simulink model "LFAST_System"  (R2022b)
settings: Solver=VariableStepAuto  StartTime=0.0  StopTime=10.0  RelTol=1e-3
model workspace (MAT data in the model file):
  LFAST_TCP_Comms = Simulink.Bus
  LFAST_TCP_Comms.Alignment = -1
  LFAST_TCP_Comms.PreserveElementDimensions = 0
  LFAST_TCP_Comms.DataScope = 'Auto'
  Modbus = Simulink.Bus
  Modbus.Alignment = -1
  Modbus.PreserveElementDimensions = 0
  Modbus.Elements_internal(1) = Simulink.BusElement
  Modbus.Elements_internal(1).DimensionsMode = 'Fixed'
  Modbus.Elements_internal(1).SamplingMode = 'Sample based'
  Modbus.Elements_internal(1).SampleTime = -1
  Modbus.Elements_internal(1).Name = 'Slave_ID'
  Modbus.Elements_internal(1).DataType_internal = 'double'
  Modbus.Elements_internal(1).Complexity = 'real'
  Modbus.Elements_internal(1).Dimensions = 1
  Modbus.Elements_internal(2) = Simulink.BusElement
  Modbus.Elements_internal(2).DimensionsMode = 'Fixed'
  Modbus.Elements_internal(2).SamplingMode = 'Sample based'
  Modbus.Elements_internal(2).SampleTime = -1
  Modbus.Elements_internal(2).Name = 'CONTROL_WORD'
  Modbus.Elements_internal(2).DataType_internal = 'double'
  Modbus.Elements_internal(2).Complexity = 'real'
  Modbus.Elements_internal(2).Dimensions = 1
  Modbus.Elements_internal(3) = Simulink.BusElement
  Modbus.Elements_internal(3).DimensionsMode = 'Fixed'
  Modbus.Elements_internal(3).SamplingMode = 'Sample based'
  Modbus.Elements_internal(3).SampleTime = -1
  Modbus.Elements_internal(3).Name = 'STATUS_WORD'
  Modbus.Elements_internal(3).DataType_internal = 'double'
  Modbus.Elements_internal(3).Complexity = 'real'
  Modbus.Elements_internal(3).Dimensions = 1
  Modbus.Elements_internal(4) = Simulink.BusElement
  Modbus.Elements_internal(4).DimensionsMode = 'Fixed'
  Modbus.Elements_internal(4).SamplingMode = 'Sample based'
  Modbus.Elements_internal(4).SampleTime = -1
  Modbus.Elements_internal(4).Name = 'OPERATION_MODE'
  Modbus.Elements_internal(4).DataType_internal = 'double'
  Modbus.Elements_internal(4).Complexity = 'real'
  Modbus.Elements_internal(4).Dimensions = 1
  Modbus.Elements_internal(5) = Simulink.BusElement
  Modbus.Elements_internal(5).DimensionsMode = 'Fixed'
  Modbus.Elements_internal(5).SamplingMode = 'Sample based'
  Modbus.Elements_internal(5).SampleTime = -1
  Modbus.Elements_internal(5).Name = 'ABS_REL_SELECT'
  Modbus.Elements_internal(5).DataType_internal = 'double'
  Modbus.Elements_internal(5).Complexity = 'real'
  Modbus.Elements_internal(5).Dimensions = 1
  Modbus.Elements_internal(6) = Simulink.BusElement
  Modbus.Elements_internal(6).DimensionsMode = 'Fixed'
  Modbus.Elements_internal(6).SamplingMode = 'Sample based'
  Modbus.Elements_internal(6).SampleTime = -1
  Modbus.Elements_internal(6).Name = 'POS_ACTUAL'
  Modbus.Elements_internal(6).DataType_internal = 'double'
  Modbus.Elements_internal(6).Complexity = 'real'
  Modbus.Elements_internal(6).Dimensions = 1
  Modbus.Elements_internal(7) = Simulink.BusElement
  Modbus.Elements_internal(7).DimensionsMode = 'Fixed'
  Modbus.Elements_internal(7).SamplingMode = 'Sample based'
  Modbus.Elements_internal(7).SampleTime = -1
  Modbus.Elements_internal(7).Name = 'REAL_CURRENT'
  Modbus.Elements_internal(7).DataType_internal = 'double'
  Modbus.Elements_internal(7).Complexity = 'real'
  Modbus.Elements_internal(7).Dimensions = 1
  Modbus.Elements_internal(8) = Simulink.BusElement
  Modbus.Elements_internal(8).DimensionsMode = 'Fixed'
  Modbus.Elements_internal(8).SamplingMode = 'Sample based'
  Modbus.Elements_internal(8).SampleTime = -1
  Modbus.Elements_internal(8).Name = 'REAL_SPEED'
  Modbus.Elements_internal(8).DataType_internal = 'double'
  Modbus.Elements_internal(8).Complexity = 'real'
  Modbus.Elements_internal(8).Dimensions = 1
  Modbus.Elements_internal(9) = Simulink.BusElement
  Modbus.Elements_internal(9).DimensionsMode = 'Fixed'
  Modbus.Elements_internal(9).SamplingMode = 'Sample based'
  Modbus.Elements_internal(9).SampleTime = -1
  Modbus.Elements_internal(9).Name = 'TARGET_POS'
  Modbus.Elements_internal(9).DataType_internal = 'double'
  Modbus.Elements_internal(9).Complexity = 'real'
  Modbus.Elements_internal(9).Dimensions = 1
  Modbus.Elements_internal(10) = Simulink.BusElement
  Modbus.Elements_internal(10).DimensionsMode = 'Fixed'
  Modbus.Elements_internal(10).SamplingMode = 'Sample based'
  Modbus.Elements_internal(10).SampleTime = -1
  Modbus.Elements_internal(10).Name = 'PROFILE_SPEED'
  Modbus.Elements_internal(10).DataType_internal = 'double'
  Modbus.Elements_internal(10).Complexity = 'real'
  Modbus.Elements_internal(10).Dimensions = 1
  Modbus.Elements_internal(11) = Simulink.BusElement
  Modbus.Elements_internal(11).DimensionsMode = 'Fixed'
  Modbus.Elements_internal(11).SamplingMode = 'Sample based'
  Modbus.Elements_internal(11).SampleTime = -1
  Modbus.Elements_internal(11).Name = 'TARGET_SPEED'
  Modbus.Elements_internal(11).DataType_internal = 'double'
  Modbus.Elements_internal(11).Complexity = 'real'
  Modbus.Elements_internal(11).Dimensions = 1
  Modbus.Elements_internal(12) = Simulink.BusElement
  Modbus.Elements_internal(12).DimensionsMode = 'Fixed'
  Modbus.Elements_internal(12).SamplingMode = 'Sample based'
  Modbus.Elements_internal(12).SampleTime = -1
  Modbus.Elements_internal(12).Name = 'MAX_SPEED'
  Modbus.Elements_internal(12).DataType_internal = 'double'
  Modbus.Elements_internal(12).Complexity = 'real'
  Modbus.Elements_internal(12).Dimensions = 1
  Modbus.Elements_internal(13) = Simulink.BusElement
  Modbus.Elements_internal(13).DimensionsMode = 'Fixed'
  Modbus.Elements_internal(13).SamplingMode = 'Sample based'
  Modbus.Elements_internal(13).SampleTime = -1
  Modbus.Elements_internal(13).Name = 'PROFILE_ACC'
  Modbus.Elements_internal(13).DataType_internal = 'double'
  Modbus.Elements_internal(13).Complexity = 'real'
  Modbus.Elements_internal(13).Dimensions = 1
  Modbus.Elements_internal(14) = Simulink.BusElement
  Modbus.Elements_internal(14).DimensionsMode = 'Fixed'
  Modbus.Elements_internal(14).SamplingMode = 'Sample based'
  Modbus.Elements_internal(14).SampleTime = -1
  Modbus.Elements_internal(14).Name = 'PROFILE_DEC'
  Modbus.Elements_internal(14).DataType_internal = 'double'
  Modbus.Elements_internal(14).Complexity = 'real'
  Modbus.Elements_internal(14).Dimensions = 1
  Modbus.Elements_internal(15) = Simulink.BusElement
  Modbus.Elements_internal(15).DimensionsMode = 'Fixed'
  Modbus.Elements_internal(15).SamplingMode = 'Sample based'
  Modbus.Elements_internal(15).SampleTime = -1
  Modbus.Elements_internal(15).Name = 'TARGET_TRQ'
  Modbus.Elements_internal(15).DataType_internal = 'double'
  Modbus.Elements_internal(15).Complexity = 'real'
  Modbus.Elements_internal(15).Dimensions = 1
  Modbus.DataScope = 'Auto'
undefined symbols (not defined in the file): AlignmentSubsystem, GuiderInterface, INDI, MessageIn, MessageOut, Telescope
settings Model: Creator=keving  LastModifiedBy=kevin
settings ModelReferenceCC: EnableRefExpFcnMdlSchedulingChecks=on

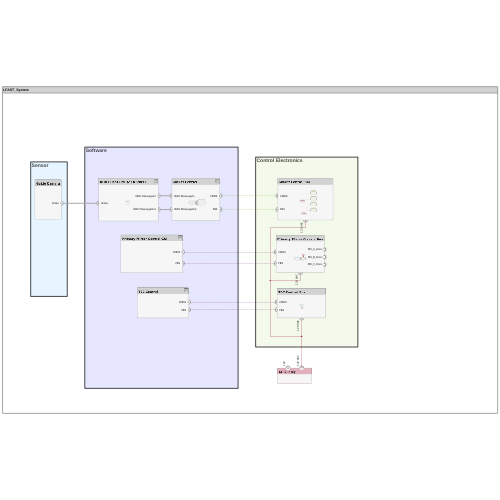
[thumbnail: Simulink's stored preview of the top-level diagram]
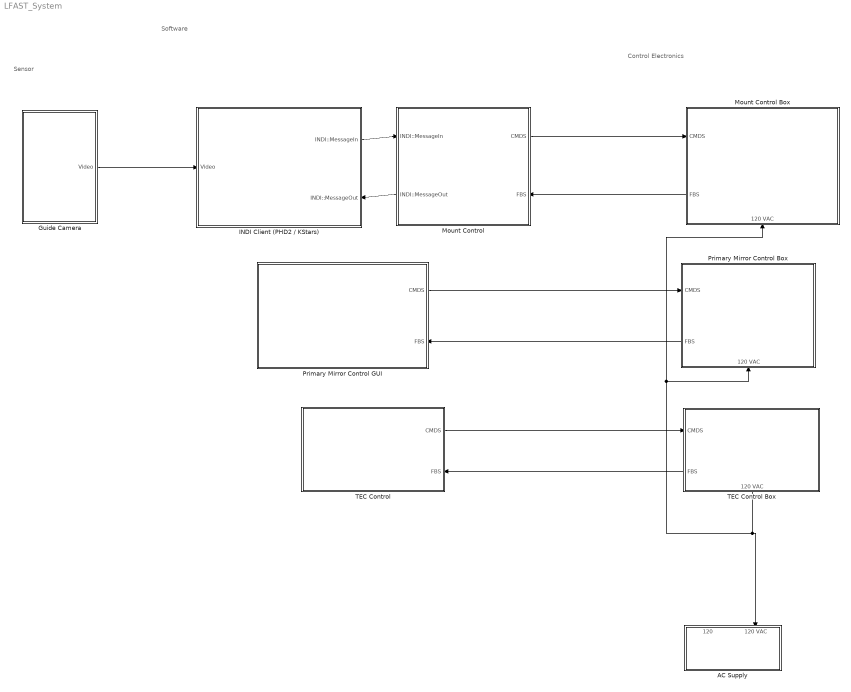
== system LFAST_System ==
  note: Sensor
  note: Software
  note: Control Electronics
  AC Supply : Subsystem
      settings: PortSchema="{\"entries\":[{\"content\":{\"headerSize\":26,\"margin\":15,\"minimumSpacing\":25,\"sides\":[{\"content\":{\"connectorIds\":[]},\"type\":\"ConnectorPlacement.EquallySpacedRectSide\",\"uuid\":\"98751f74-1494-480e-afcb-1e4ca4833d8c\"},{\"content\":{\"connectorIds\":[],\"side\":\"RIGHT\"},\"type\":\"ConnectorPlacement.EquallySpacedRectSide\",\"uuid\":\"bb8add54-8697-4b5a-a683-6c55bc29b1b0\"},{\"content\":{\"connectorIds\":[\"Out1\",\"In1\"],\"side\":\"TOP\"},\"type\":\"ConnectorPlacement.EquallySpacedRectSide\",\"uuid\":\"300d0c82-b670-4163-bf95-251aaf6b9511\"},{\"content\":{\"connectorIds\":[],\"side\":\"BOTTOM\"},\"type\":\"ConnectorPlacement.EquallySpacedRectSide\",\"uuid\":\"167ec2d4-c810-4164-afac-a7cf55661aff\"}]},\"type\":\"ConnectorPlacement.EquallySpacedConnector\",\"uuid\":\"bf69df94-f6ab-4503-8752-ba9a09e2aadb\"}],\"packageUris\":[\"http://schema.mathworks.com/mf0/Connector/R2020b\"],\"version\":\"1.0\"}"
  Guide Camera : Subsystem
      settings: PortSchema="{\"entries\":[{\"content\":{\"headerSize\":26,\"margin\":15,\"minimumSpacing\":25,\"sides\":[{\"content\":{\"connectorIds\":[]},\"type\":\"ConnectorPlacement.EquallySpacedRectSide\",\"uuid\":\"16df8581-7966-4d2c-895b-cc4ea5e246e2\"},{\"content\":{\"connectorIds\":[\"Out1\"],\"side\":\"RIGHT\"},\"type\":\"ConnectorPlacement.EquallySpacedRectSide\",\"uuid\":\"5d59704d-ff3e-44f0-a7f2-847c95827cea\"},{\"content\":{\"connectorIds\":[],\"side\":\"TOP\"},\"type\":\"ConnectorPlacement.EquallySpacedRectSide\",\"uuid\":\"ec3ed101-a96e-4d79-89e3-2afa312ea215\"}]},\"type\":\"ConnectorPlacement.EquallySpacedConnector\",\"uuid\":\"5d368a71-4eba-4adc-b01b-0abb6bcb9ebc\"}],\"packageUris\":[\"http://schema.mathworks.com/mf0/Connector/R2020b\"],\"version\":\"1.0\"}"
  INDI Client (PHD2 / KStars) : Subsystem
      settings: PortSchema="{\"entries\":[{\"content\":{\"headerSize\":26,\"margin\":15,\"minimumSpacing\":25,\"sides\":[{\"content\":{\"connectorIds\":[\"In1\"]},\"type\":\"ConnectorPlacement.EquallySpacedRectSide\",\"uuid\":\"1ee64d24-9451-4e89-96b0-c6c86ed53331\"},{\"content\":{\"connectorIds\":[\"Out1\",\"In2\"],\"side\":\"RIGHT\"},\"type\":\"ConnectorPlacement.EquallySpacedRectSide\",\"uuid\":\"58644688-a0cb-4784-bb9d-85cd24f76786\"},{\"content\":{\"connectorIds\":[],\"side\":\"TOP\"},\"type\":\"ConnectorPlacement.EquallySpacedRectSide\",\"uuid\":\"73e421bb-b1b1-4cf2-a19d-6b2642b6c763\"},{\"content\":{\"connectorIds\":[],\"side\":\"BOTTOM\"},\"type\":\"ConnectorPlacement.EquallySpacedRectSide\",\"uuid\":\"a1df0027-ba85-456a-a33c-a4e3aae0142d\"}]},\"type\":\"ConnectorPlacement.EquallySpacedConnector\",\"uuid\":\"5578c5ac-9f78-4996-ba84-f029b9b17e19\"}],\"packageUris\":[\"http://schema.mathworks.com/mf0/Connector/R2020b\"],\"version\":\"1.0\"}"
  Mount Control : Subsystem
      settings: PortSchema="{\"entries\":[{\"content\":{\"headerSize\":26,\"margin\":15,\"minimumSpacing\":25,\"sides\":[{\"content\":{\"connectorIds\":[\"In2\",\"Out2\"]},\"type\":\"ConnectorPlacement.EquallySpacedRectSide\",\"uuid\":\"1e7a6f7e-04b1-487d-9c42-3f004f45fff7\"},{\"content\":{\"connectorIds\":[\"Out1\",\"In1\"],\"side\":\"RIGHT\"},\"type\":\"ConnectorPlacement.EquallySpacedRectSide\",\"uuid\":\"1d40cd5a-d50e-48bb-ba62-29f418ee0b7d\"},{\"content\":{\"connectorIds\":[],\"side\":\"TOP\"},\"type\":\"ConnectorPlacement.EquallySpacedRectSide\",\"uuid\":\"8c60b213-5e96-4c1f-bace-a9a184d6d43c\"},{\"content\":{\"connectorIds\":[],\"side\":\"BOTTOM\"},\"type\":\"ConnectorPlacement.EquallySpacedRectSide\",\"uuid\":\"7f5ded68-ba2c-42b9-9d6b-2756d3ededc8\"}]},\"type\":\"ConnectorPlacement.EquallySpacedConnector\",\"uuid\":\"740ba7aa-7f0b-4fdf-8ac9-38c1be24b304\"}],\"packageUris\":[\"http://schema.mathworks.com/mf0/Connector/R2020b\"],\"version\":\"1.0\"}"
  Mount Control Box : Subsystem
      settings: PortSchema="{\"entries\":[{\"content\":{\"headerSize\":26,\"margin\":15,\"minimumSpacing\":25,\"sides\":[{\"content\":{\"connectorIds\":[\"In2\",\"Out1\"]},\"type\":\"ConnectorPlacement.EquallySpacedRectSide\",\"uuid\":\"16df8581-7966-4d2c-895b-cc4ea5e246e2\"},{\"content\":{\"connectorIds\":[],\"side\":\"RIGHT\"},\"type\":\"ConnectorPlacement.EquallySpacedRectSide\",\"uuid\":\"5d59704d-ff3e-44f0-a7f2-847c95827cea\"},{\"content\":{\"connectorIds\":[],\"side\":\"TOP\"},\"type\":\"ConnectorPlacement.EquallySpacedRectSide\",\"uuid\":\"ec3ed101-a96e-4d79-89e3-2afa312ea215\"},{\"content\":{\"connectorIds\":[\"In1\"],\"side\":\"BOTTOM\"},\"type\":\"ConnectorPlacement.EquallySpacedRectSide\",\"uuid\":\"65d70669-a716-492b-bf91-097d7de9987f\"}]},\"type\":\"ConnectorPlacement.EquallySpacedConnector\",\"uuid\":\"5d368a71-4eba-4adc-b01b-0abb6bcb9ebc\"}],\"packageUris\":[\"http://schema.mathworks.com/mf0/Connector/R2020b\"],\"version\":\"1.0\"}"
  Primary Mirror Control Box : Subsystem
      settings: PortSchema="{\"entries\":[{\"content\":{\"headerSize\":26,\"margin\":15,\"minimumSpacing\":25,\"sides\":[{\"content\":{\"connectorIds\":[\"In2\",\"Out1\"]},\"type\":\"ConnectorPlacement.EquallySpacedRectSide\",\"uuid\":\"8068dc4f-e0e9-4f1b-946a-b531e46fc784\"},{\"content\":{\"connectorIds\":[\"RConn1\",\"RConn2\",\"RConn3\"],\"side\":\"RIGHT\"},\"type\":\"ConnectorPlacement.EquallySpacedRectSide\",\"uuid\":\"7b44236b-1168-43b8-b2b4-5e873209dfa3\"},{\"content\":{\"connectorIds\":[],\"side\":\"TOP\"},\"type\":\"ConnectorPlacement.EquallySpacedRectSide\",\"uuid\":\"fca4122f-6519-48a9-876a-2e597a8d3bc7\"},{\"content\":{\"connectorIds\":[\"In1\"],\"side\":\"BOTTOM\"},\"type\":\"ConnectorPlacement.EquallySpacedRectSide\",\"uuid\":\"6f4aa163-7b47-4691-94b1-15c4b7706454\"}]},\"type\":\"ConnectorPlacement.EquallySpacedConnector\",\"uuid\":\"9787fa30-fe20-4a09-9d69-8b8b4a760450\"}],\"packageUris\":[\"http://schema.mathworks.com/mf0/Connector/R2020b\"],\"version\":\"1.0\"}"
  Primary Mirror Control GUI : Subsystem
      settings: PortSchema="{\"entries\":[{\"content\":{\"headerSize\":26,\"margin\":15,\"minimumSpacing\":25,\"sides\":[{\"content\":{\"connectorIds\":[]},\"type\":\"ConnectorPlacement.EquallySpacedRectSide\",\"uuid\":\"98751f74-1494-480e-afcb-1e4ca4833d8c\"},{\"content\":{\"connectorIds\":[\"Out1\",\"In1\"],\"side\":\"RIGHT\"},\"type\":\"ConnectorPlacement.EquallySpacedRectSide\",\"uuid\":\"bb8add54-8697-4b5a-a683-6c55bc29b1b0\"},{\"content\":{\"connectorIds\":[],\"side\":\"TOP\"},\"type\":\"ConnectorPlacement.EquallySpacedRectSide\",\"uuid\":\"300d0c82-b670-4163-bf95-251aaf6b9511\"},{\"content\":{\"connectorIds\":[],\"side\":\"BOTTOM\"},\"type\":\"ConnectorPlacement.EquallySpacedRectSide\",\"uuid\":\"da416aef-0667-4671-a4f6-786b74bf3980\"}]},\"type\":\"ConnectorPlacement.EquallySpacedConnector\",\"uuid\":\"bf69df94-f6ab-4503-8752-ba9a09e2aadb\"}],\"packageUris\":[\"http://schema.mathworks.com/mf0/Connector/R2020b\"],\"version\":\"1.0\"}"
  TEC Control : Subsystem
      settings: PortSchema="{\"entries\":[{\"content\":{\"headerSize\":26,\"margin\":15,\"minimumSpacing\":25,\"sides\":[{\"content\":{\"connectorIds\":[]},\"type\":\"ConnectorPlacement.EquallySpacedRectSide\",\"uuid\":\"98751f74-1494-480e-afcb-1e4ca4833d8c\"},{\"content\":{\"connectorIds\":[\"Out1\",\"In1\"],\"side\":\"RIGHT\"},\"type\":\"ConnectorPlacement.EquallySpacedRectSide\",\"uuid\":\"bb8add54-8697-4b5a-a683-6c55bc29b1b0\"},{\"content\":{\"connectorIds\":[],\"side\":\"TOP\"},\"type\":\"ConnectorPlacement.EquallySpacedRectSide\",\"uuid\":\"300d0c82-b670-4163-bf95-251aaf6b9511\"}]},\"type\":\"ConnectorPlacement.EquallySpacedConnector\",\"uuid\":\"bf69df94-f6ab-4503-8752-ba9a09e2aadb\"}],\"packageUris\":[\"http://schema.mathworks.com/mf0/Connector/R2020b\"],\"version\":\"1.0\"}"
  TEC Control Box : Subsystem
      settings: PortSchema="{\"entries\":[{\"content\":{\"headerSize\":26,\"margin\":15,\"minimumSpacing\":25,\"sides\":[{\"content\":{\"connectorIds\":[\"In1\",\"Out2\"]},\"type\":\"ConnectorPlacement.EquallySpacedRectSide\",\"uuid\":\"8068dc4f-e0e9-4f1b-946a-b531e46fc784\"},{\"content\":{\"connectorIds\":[],\"side\":\"RIGHT\"},\"type\":\"ConnectorPlacement.EquallySpacedRectSide\",\"uuid\":\"7b44236b-1168-43b8-b2b4-5e873209dfa3\"},{\"content\":{\"connectorIds\":[],\"side\":\"TOP\"},\"type\":\"ConnectorPlacement.EquallySpacedRectSide\",\"uuid\":\"fca4122f-6519-48a9-876a-2e597a8d3bc7\"},{\"content\":{\"connectorIds\":[\"Out1\"],\"side\":\"BOTTOM\"},\"type\":\"ConnectorPlacement.EquallySpacedRectSide\",\"uuid\":\"c7e8194f-a12b-4ae8-b7ba-58203e5e8cbe\"}]},\"type\":\"ConnectorPlacement.EquallySpacedConnector\",\"uuid\":\"9787fa30-fe20-4a09-9d69-8b8b4a760450\"}],\"packageUris\":[\"http://schema.mathworks.com/mf0/Connector/R2020b\"],\"version\":\"1.0\"}"
  wires:
  INDI Client (PHD2 / KStars)/1(INDI::MessageIn) -> Mount Control/2(INDI::MessageIn)
  Mount Control/2(INDI::MessageOut) -> INDI Client (PHD2 / KStars)/2(INDI::MessageOut)
  Guide Camera/1(Video) -> INDI Client (PHD2 / KStars)/1(Video)
  Mount Control/1(CMDS) -> Mount Control Box/2(CMDS)
  Mount Control Box/1(FBS) -> Mount Control/1(FBS)
  Primary Mirror Control GUI/1(CMDS) -> Primary Mirror Control Box/2(CMDS)
  Primary Mirror Control Box/1(FBS) -> Primary Mirror Control GUI/1(FBS)
  TEC Control/1(CMDS) -> TEC Control Box/1(CMDS)
  TEC Control Box/2(FBS) -> TEC Control/1(FBS)
  TEC Control Box/1(120 VAC) -> Mount Control Box/1(120 VAC), Primary Mirror Control Box/1(120 VAC), AC Supply/1(120 VAC)

== system LFAST_System/AC Supply ==
  Bus Element In1 : Inport  PortName=120 VAC
  Bus Element Out1 : Outport  PortName=120

== system LFAST_System/Guide Camera ==
  Bus Element Out1 : Outport  PortName=Video

== system LFAST_System/INDI Client (PHD2 // KStars) ==
  Bus Element In3 : Inport  PortName=Video
  Bus Element In2 : Inport  Port=2  PortName=INDI::MessageOut
  Plate Solver : Subsystem
      settings: PortSchema="{\"entries\":[{\"content\":{\"headerSize\":26,\"margin\":15,\"minimumSpacing\":25,\"sides\":[{\"content\":{\"connectorIds\":[]},\"type\":\"ConnectorPlacement.EquallySpacedRectSide\",\"uuid\":\"308388c6-8e91-479e-9011-1f7a7fcb1cce\"},{\"content\":{\"connectorIds\":[],\"side\":\"RIGHT\"},\"type\":\"ConnectorPlacement.EquallySpacedRectSide\",\"uuid\":\"7c8e7e56-15f1-4cfc-9de2-99c590c1d901\"},{\"content\":{\"connectorIds\":[],\"side\":\"TOP\"},\"type\":\"ConnectorPlacement.EquallySpacedRectSide\",\"uuid\":\"16936ed8-c29c-40e6-ab62-02c7d1bd68c4\"}]},\"type\":\"ConnectorPlacement.EquallySpacedConnector\",\"uuid\":\"eb7df44b-8d85-4bd6-b6b8-056a4c77b10a\"}],\"packageUris\":[\"http://schema.mathworks.com/mf0/Connector/R2020b\"],\"version\":\"1.0\"}"
  Bus Element Out1 : Outport  PortName=INDI::MessageIn

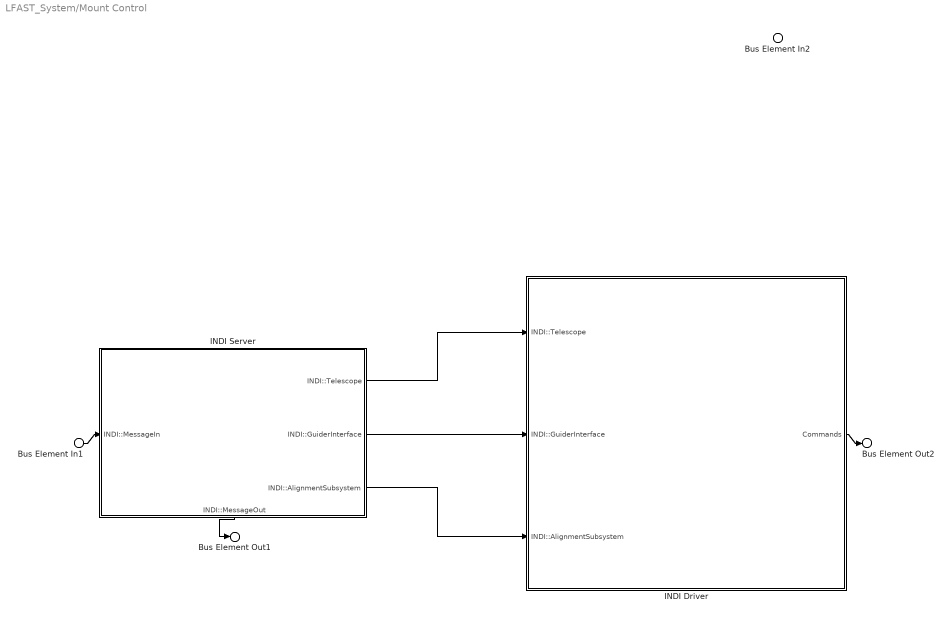
== system LFAST_System/Mount Control ==
  Bus Element In2 : Inport  PortName=FBS
  Bus Element In1 : Inport  Port=2  PortName=INDI::MessageIn
  INDI Driver : Subsystem
      settings: PortSchema="{\"entries\":[{\"content\":{\"headerSize\":26,\"margin\":15,\"minimumSpacing\":25,\"sides\":[{\"content\":{\"connectorIds\":[\"In1\",\"In2\",\"In3\"]},\"type\":\"ConnectorPlacement.EquallySpacedRectSide\",\"uuid\":\"84fd24e3-afcf-4794-b886-f32f0ca70f22\"},{\"content\":{\"connectorIds\":[\"Out1\"],\"side\":\"RIGHT\"},\"type\":\"ConnectorPlacement.EquallySpacedRectSide\",\"uuid\":\"ce034fd2-72c0-4e78-b116-46e515910606\"},{\"content\":{\"connectorIds\":[],\"side\":\"TOP\"},\"type\":\"ConnectorPlacement.EquallySpacedRectSide\",\"uuid\":\"d1df9167-d909-40fe-8e6c-af454ddadc5a\"},{\"content\":{\"connectorIds\":[],\"side\":\"BOTTOM\"},\"type\":\"ConnectorPlacement.EquallySpacedRectSide\",\"uuid\":\"ee59ff0f-8052-43a5-a6ea-649f12a036f7\"}]},\"type\":\"ConnectorPlacement.EquallySpacedConnector\",\"uuid\":\"aa2eec28-162c-47d7-923d-9f626bd6b64a\"}],\"packageUris\":[\"http://schema.mathworks.com/mf0/Connector/R2020b\"],\"version\":\"1.0\"}"
  INDI Server : Subsystem
      settings: PortSchema="{\"entries\":[{\"content\":{\"headerSize\":26,\"margin\":15,\"minimumSpacing\":25,\"sides\":[{\"content\":{\"connectorIds\":[\"In1\"]},\"type\":\"ConnectorPlacement.EquallySpacedRectSide\",\"uuid\":\"3de6b7f9-ed8a-45a6-8468-10e2cec44851\"},{\"content\":{\"connectorIds\":[\"Out2\",\"Out3\",\"Out4\"],\"side\":\"RIGHT\"},\"type\":\"ConnectorPlacement.EquallySpacedRectSide\",\"uuid\":\"2f599830-52f9-4db6-bde0-76538885e5e3\"},{\"content\":{\"connectorIds\":[],\"side\":\"TOP\"},\"type\":\"ConnectorPlacement.EquallySpacedRectSide\",\"uuid\":\"800350c6-ea2c-4543-8788-57b5fa38085a\"},{\"content\":{\"connectorIds\":[\"Out1\"],\"side\":\"BOTTOM\"},\"type\":\"ConnectorPlacement.EquallySpacedRectSide\",\"uuid\":\"129328fe-34d5-4d45-bd17-bced5dbfaccb\"}]},\"type\":\"ConnectorPlacement.EquallySpacedConnector\",\"uuid\":\"5cda8e6f-f3f0-4ed4-a17f-f9ee45db8f44\"}],\"packageUris\":[\"http://schema.mathworks.com/mf0/Connector/R2020b\"],\"version\":\"1.0\"}"
  Bus Element Out2 : Outport  PortName=CMDS
  Bus Element Out1 : Outport  Port=2  PortName=INDI::MessageOut
  wires:
  INDI Server/2(INDI::Telescope) -> INDI Driver/1(INDI::Telescope)
  INDI Server/3(INDI::GuiderInterface) -> INDI Driver/2(INDI::GuiderInterface)
  INDI Server/4(INDI::AlignmentSubsystem) -> INDI Driver/3(INDI::AlignmentSubsystem)
  INDI Driver/1(Commands) -> Bus Element Out2/1
  INDI Server/1(INDI::MessageOut) -> Bus Element Out1/1
  Bus Element In1/1 -> INDI Server/1(INDI::MessageIn)

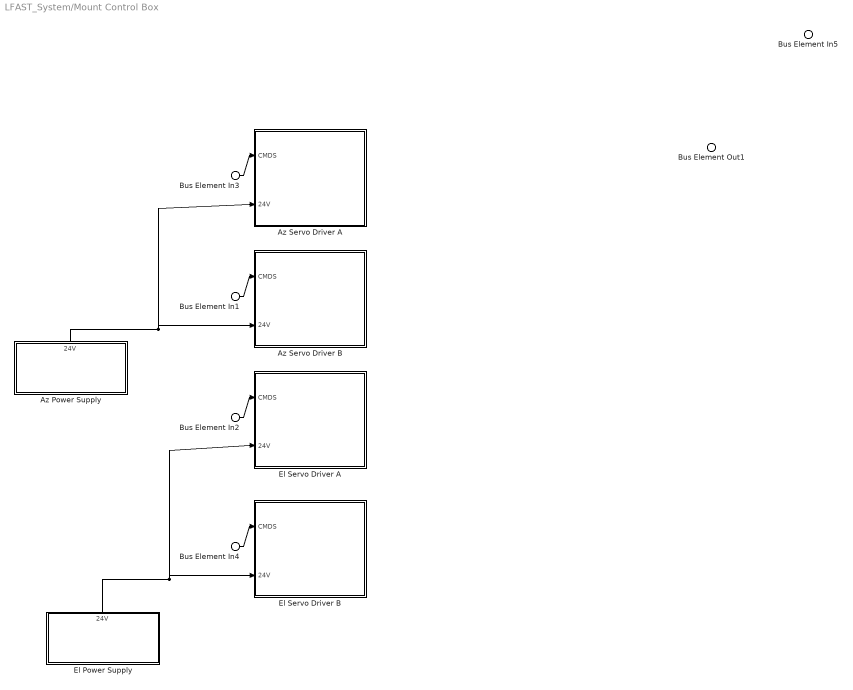
== system LFAST_System/Mount Control Box ==
  Bus Element In5 : Inport  PortName=120 VAC
  Bus Element In{1..4} (4 alike) : Inport  Port=2  PortName=CMDS
  Az Power Supply : Subsystem
      settings: PortSchema="{\"entries\":[{\"content\":{\"headerSize\":26,\"margin\":15,\"minimumSpacing\":25,\"sides\":[{\"content\":{\"connectorIds\":[]},\"type\":\"ConnectorPlacement.EquallySpacedRectSide\",\"uuid\":\"98751f74-1494-480e-afcb-1e4ca4833d8c\"},{\"content\":{\"connectorIds\":[],\"side\":\"RIGHT\"},\"type\":\"ConnectorPlacement.EquallySpacedRectSide\",\"uuid\":\"bb8add54-8697-4b5a-a683-6c55bc29b1b0\"},{\"content\":{\"connectorIds\":[\"Out1\"],\"side\":\"TOP\"},\"type\":\"ConnectorPlacement.EquallySpacedRectSide\",\"uuid\":\"300d0c82-b670-4163-bf95-251aaf6b9511\"},{\"content\":{\"connectorIds\":[],\"side\":\"BOTTOM\"},\"type\":\"ConnectorPlacement.EquallySpacedRectSide\",\"uuid\":\"167ec2d4-c810-4164-afac-a7cf55661aff\"}]},\"type\":\"ConnectorPlacement.EquallySpacedConnector\",\"uuid\":\"bf69df94-f6ab-4503-8752-ba9a09e2aadb\"}],\"packageUris\":[\"http://schema.mathworks.com/mf0/Connector/R2020b\"],\"version\":\"1.0\"}"
  Az Servo Driver A : Subsystem
      settings: PortSchema="{\"entries\":[{\"content\":{\"headerSize\":26,\"margin\":15,\"minimumSpacing\":25,\"sides\":[{\"content\":{\"connectorIds\":[\"In1\",\"In2\"]},\"type\":\"ConnectorPlacement.EquallySpacedRectSide\",\"uuid\":\"16df8581-7966-4d2c-895b-cc4ea5e246e2\"},{\"content\":{\"connectorIds\":[\"RConn1\",\"RConn2\",\"RConn3\"],\"side\":\"RIGHT\"},\"type\":\"ConnectorPlacement.EquallySpacedRectSide\",\"uuid\":\"5d59704d-ff3e-44f0-a7f2-847c95827cea\"},{\"content\":{\"connectorIds\":[],\"side\":\"TOP\"},\"type\":\"ConnectorPlacement.EquallySpacedRectSide\",\"uuid\":\"ec3ed101-a96e-4d79-89e3-2afa312ea215\"}]},\"type\":\"ConnectorPlacement.EquallySpacedConnector\",\"uuid\":\"5d368a71-4eba-4adc-b01b-0abb6bcb9ebc\"}],\"packageUris\":[\"http://schema.mathworks.com/mf0/Connector/R2020b\"],\"version\":\"1.0\"}"
  Az Servo Driver B : Subsystem
      settings: PortSchema="{\"entries\":[{\"content\":{\"headerSize\":26,\"margin\":15,\"minimumSpacing\":25,\"sides\":[{\"content\":{\"connectorIds\":[\"In1\",\"In2\"]},\"type\":\"ConnectorPlacement.EquallySpacedRectSide\",\"uuid\":\"16df8581-7966-4d2c-895b-cc4ea5e246e2\"},{\"content\":{\"connectorIds\":[\"RConn1\",\"RConn2\",\"RConn3\"],\"side\":\"RIGHT\"},\"type\":\"ConnectorPlacement.EquallySpacedRectSide\",\"uuid\":\"5d59704d-ff3e-44f0-a7f2-847c95827cea\"},{\"content\":{\"connectorIds\":[],\"side\":\"TOP\"},\"type\":\"ConnectorPlacement.EquallySpacedRectSide\",\"uuid\":\"ec3ed101-a96e-4d79-89e3-2afa312ea215\"}]},\"type\":\"ConnectorPlacement.EquallySpacedConnector\",\"uuid\":\"5d368a71-4eba-4adc-b01b-0abb6bcb9ebc\"}],\"packageUris\":[\"http://schema.mathworks.com/mf0/Connector/R2020b\"],\"version\":\"1.0\"}"
  El Power Supply : Subsystem
      settings: PortSchema="{\"entries\":[{\"content\":{\"headerSize\":26,\"margin\":15,\"minimumSpacing\":25,\"sides\":[{\"content\":{\"connectorIds\":[]},\"type\":\"ConnectorPlacement.EquallySpacedRectSide\",\"uuid\":\"98751f74-1494-480e-afcb-1e4ca4833d8c\"},{\"content\":{\"connectorIds\":[],\"side\":\"RIGHT\"},\"type\":\"ConnectorPlacement.EquallySpacedRectSide\",\"uuid\":\"bb8add54-8697-4b5a-a683-6c55bc29b1b0\"},{\"content\":{\"connectorIds\":[\"Out1\"],\"side\":\"TOP\"},\"type\":\"ConnectorPlacement.EquallySpacedRectSide\",\"uuid\":\"300d0c82-b670-4163-bf95-251aaf6b9511\"},{\"content\":{\"connectorIds\":[],\"side\":\"BOTTOM\"},\"type\":\"ConnectorPlacement.EquallySpacedRectSide\",\"uuid\":\"167ec2d4-c810-4164-afac-a7cf55661aff\"}]},\"type\":\"ConnectorPlacement.EquallySpacedConnector\",\"uuid\":\"bf69df94-f6ab-4503-8752-ba9a09e2aadb\"}],\"packageUris\":[\"http://schema.mathworks.com/mf0/Connector/R2020b\"],\"version\":\"1.0\"}"
  El Servo Driver A : Subsystem
      settings: PortSchema="{\"entries\":[{\"content\":{\"headerSize\":26,\"margin\":15,\"minimumSpacing\":25,\"sides\":[{\"content\":{\"connectorIds\":[\"In1\",\"In2\"]},\"type\":\"ConnectorPlacement.EquallySpacedRectSide\",\"uuid\":\"16df8581-7966-4d2c-895b-cc4ea5e246e2\"},{\"content\":{\"connectorIds\":[\"RConn1\",\"RConn2\",\"RConn3\"],\"side\":\"RIGHT\"},\"type\":\"ConnectorPlacement.EquallySpacedRectSide\",\"uuid\":\"5d59704d-ff3e-44f0-a7f2-847c95827cea\"},{\"content\":{\"connectorIds\":[],\"side\":\"TOP\"},\"type\":\"ConnectorPlacement.EquallySpacedRectSide\",\"uuid\":\"ec3ed101-a96e-4d79-89e3-2afa312ea215\"}]},\"type\":\"ConnectorPlacement.EquallySpacedConnector\",\"uuid\":\"5d368a71-4eba-4adc-b01b-0abb6bcb9ebc\"}],\"packageUris\":[\"http://schema.mathworks.com/mf0/Connector/R2020b\"],\"version\":\"1.0\"}"
  El Servo Driver B : Subsystem
      settings: PortSchema="{\"entries\":[{\"content\":{\"headerSize\":26,\"margin\":15,\"minimumSpacing\":25,\"sides\":[{\"content\":{\"connectorIds\":[\"In1\",\"In2\"]},\"type\":\"ConnectorPlacement.EquallySpacedRectSide\",\"uuid\":\"16df8581-7966-4d2c-895b-cc4ea5e246e2\"},{\"content\":{\"connectorIds\":[\"RConn1\",\"RConn2\",\"RConn3\"],\"side\":\"RIGHT\"},\"type\":\"ConnectorPlacement.EquallySpacedRectSide\",\"uuid\":\"5d59704d-ff3e-44f0-a7f2-847c95827cea\"},{\"content\":{\"connectorIds\":[],\"side\":\"TOP\"},\"type\":\"ConnectorPlacement.EquallySpacedRectSide\",\"uuid\":\"ec3ed101-a96e-4d79-89e3-2afa312ea215\"}]},\"type\":\"ConnectorPlacement.EquallySpacedConnector\",\"uuid\":\"5d368a71-4eba-4adc-b01b-0abb6bcb9ebc\"}],\"packageUris\":[\"http://schema.mathworks.com/mf0/Connector/R2020b\"],\"version\":\"1.0\"}"
  Bus Element Out1 : Outport  PortName=FBS
  wires:
  Az Power Supply/1(24V) -> Az Servo Driver B/2(24V), Az Servo Driver A/2(24V)
  El Power Supply/1(24V) -> El Servo Driver A/2(24V), El Servo Driver B/2(24V)
  Bus Element In3/1 -> Az Servo Driver A/1(CMDS)
  Bus Element In1/1 -> Az Servo Driver B/1(CMDS)
  Bus Element In2/1 -> El Servo Driver A/1(CMDS)
  Bus Element In4/1 -> El Servo Driver B/1(CMDS)

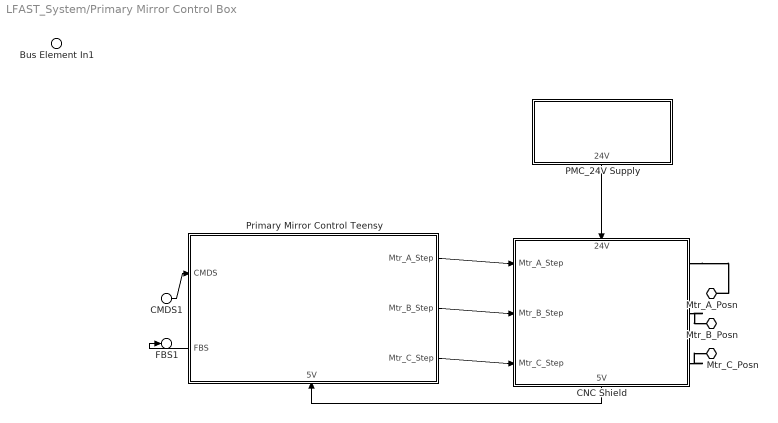
== system LFAST_System/Primary Mirror Control Box ==
  Bus Element In1 : Inport  PortName=120 VAC
  CMDS1 : Inport  Port=2  PortName=CMDS
  CNC Shield : Subsystem
      settings: PortSchema="{\"entries\":[{\"content\":{\"headerSize\":26,\"margin\":15,\"minimumSpacing\":25,\"sides\":[{\"content\":{\"connectorIds\":[\"In2\",\"In3\",\"In4\"]},\"type\":\"ConnectorPlacement.EquallySpacedRectSide\",\"uuid\":\"98751f74-1494-480e-afcb-1e4ca4833d8c\"},{\"content\":{\"connectorIds\":[\"RConn1\",\"RConn2\",\"RConn3\"],\"side\":\"RIGHT\"},\"type\":\"ConnectorPlacement.EquallySpacedRectSide\",\"uuid\":\"bb8add54-8697-4b5a-a683-6c55bc29b1b0\"},{\"content\":{\"connectorIds\":[\"In1\"],\"side\":\"TOP\"},\"type\":\"ConnectorPlacement.EquallySpacedRectSide\",\"uuid\":\"300d0c82-b670-4163-bf95-251aaf6b9511\"},{\"content\":{\"connectorIds\":[\"Out1\"],\"side\":\"BOTTOM\"},\"type\":\"ConnectorPlacement.EquallySpacedRectSide\",\"uuid\":\"6e75f32b-8584-4281-a5db-600f708f169a\"}]},\"type\":\"ConnectorPlacement.EquallySpacedConnector\",\"uuid\":\"bf69df94-f6ab-4503-8752-ba9a09e2aadb\"}],\"packageUris\":[\"http://schema.mathworks.com/mf0/Connector/R2020b\"],\"version\":\"1.0\"}"
  PMC_24V Supply : Subsystem
      settings: PortSchema="{\"entries\":[{\"content\":{\"headerSize\":26,\"margin\":15,\"minimumSpacing\":25,\"sides\":[{\"content\":{\"connectorIds\":[]},\"type\":\"ConnectorPlacement.EquallySpacedRectSide\",\"uuid\":\"98751f74-1494-480e-afcb-1e4ca4833d8c\"},{\"content\":{\"connectorIds\":[],\"side\":\"RIGHT\"},\"type\":\"ConnectorPlacement.EquallySpacedRectSide\",\"uuid\":\"bb8add54-8697-4b5a-a683-6c55bc29b1b0\"},{\"content\":{\"connectorIds\":[],\"side\":\"TOP\"},\"type\":\"ConnectorPlacement.EquallySpacedRectSide\",\"uuid\":\"300d0c82-b670-4163-bf95-251aaf6b9511\"},{\"content\":{\"connectorIds\":[\"Out1\"],\"side\":\"BOTTOM\"},\"type\":\"ConnectorPlacement.EquallySpacedRectSide\",\"uuid\":\"167ec2d4-c810-4164-afac-a7cf55661aff\"}]},\"type\":\"ConnectorPlacement.EquallySpacedConnector\",\"uuid\":\"bf69df94-f6ab-4503-8752-ba9a09e2aadb\"}],\"packageUris\":[\"http://schema.mathworks.com/mf0/Connector/R2020b\"],\"version\":\"1.0\"}"
  Primary Mirror Control Teensy : Subsystem
      settings: PortSchema="{\"entries\":[{\"content\":{\"headerSize\":26,\"margin\":15,\"minimumSpacing\":25,\"sides\":[{\"content\":{\"connectorIds\":[\"In2\",\"Out4\"]},\"type\":\"ConnectorPlacement.EquallySpacedRectSide\",\"uuid\":\"98751f74-1494-480e-afcb-1e4ca4833d8c\"},{\"content\":{\"connectorIds\":[\"Out1\",\"Out2\",\"Out3\"],\"side\":\"RIGHT\"},\"type\":\"ConnectorPlacement.EquallySpacedRectSide\",\"uuid\":\"bb8add54-8697-4b5a-a683-6c55bc29b1b0\"},{\"content\":{\"connectorIds\":[],\"side\":\"TOP\"},\"type\":\"ConnectorPlacement.EquallySpacedRectSide\",\"uuid\":\"300d0c82-b670-4163-bf95-251aaf6b9511\"},{\"content\":{\"connectorIds\":[\"In1\"],\"side\":\"BOTTOM\"},\"type\":\"ConnectorPlacement.EquallySpacedRectSide\",\"uuid\":\"8a75bd41-e78c-494e-8047-06aa70d42565\"}]},\"type\":\"ConnectorPlacement.EquallySpacedConnector\",\"uuid\":\"bf69df94-f6ab-4503-8752-ba9a09e2aadb\"}],\"packageUris\":[\"http://schema.mathworks.com/mf0/Connector/R2020b\"],\"version\":\"1.0\"}"
  Mtr_A_Posn : PMIOPort  Side=Right
  Mtr_B_Posn : PMIOPort  Port=2  Side=Right
  Mtr_C_Posn : PMIOPort  Port=3  Side=Right
  FBS1 : Outport  PortName=FBS
  wires:
  Primary Mirror Control Teensy/2(Mtr_B_Step) -> CNC Shield/3(Mtr_B_Step)
  Primary Mirror Control Teensy/1(Mtr_A_Step) -> CNC Shield/2(Mtr_A_Step)
  PMC_24V Supply/1(24V) -> CNC Shield/1(24V)
  Primary Mirror Control Teensy/3(Mtr_C_Step) -> CNC Shield/4(Mtr_C_Step)
  CNC Shield/1(5V) -> Primary Mirror Control Teensy/1(5V)
  Primary Mirror Control Teensy/4(FBS) -> FBS1/1
  CMDS1/1 -> Primary Mirror Control Teensy/2(CMDS)
  connections:
  CNC Shield/RConn1 -- Mtr_A_Posn/RConn1
  CNC Shield/RConn2 -- Mtr_B_Posn/RConn1
  CNC Shield/RConn3 -- Mtr_C_Posn/RConn1

== system LFAST_System/Primary Mirror Control GUI ==
  Bus Element In1 : Inport  PortName=FBS
  Bus Element Out1 : Outport  PortName=CMDS

== system LFAST_System/TEC Control ==
  Bus Element In1 : Inport  PortName=FBS
  Bus Element Out1 : Outport  PortName=CMDS

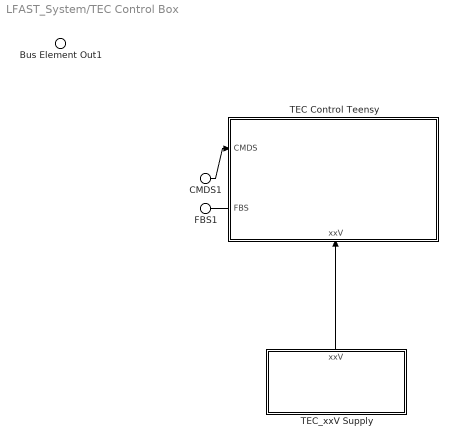
== system LFAST_System/TEC Control Box ==
  CMDS1 : Inport  PortName=CMDS
  TEC Control Teensy : Subsystem
      settings: PortSchema="{\"entries\":[{\"content\":{\"headerSize\":26,\"margin\":15,\"minimumSpacing\":25,\"sides\":[{\"content\":{\"connectorIds\":[\"In2\",\"Out1\"]},\"type\":\"ConnectorPlacement.EquallySpacedRectSide\",\"uuid\":\"98751f74-1494-480e-afcb-1e4ca4833d8c\"},{\"content\":{\"connectorIds\":[],\"side\":\"RIGHT\"},\"type\":\"ConnectorPlacement.EquallySpacedRectSide\",\"uuid\":\"bb8add54-8697-4b5a-a683-6c55bc29b1b0\"},{\"content\":{\"connectorIds\":[],\"side\":\"TOP\"},\"type\":\"ConnectorPlacement.EquallySpacedRectSide\",\"uuid\":\"300d0c82-b670-4163-bf95-251aaf6b9511\"},{\"content\":{\"connectorIds\":[\"In1\"],\"side\":\"BOTTOM\"},\"type\":\"ConnectorPlacement.EquallySpacedRectSide\",\"uuid\":\"30694b7a-2b9c-40e9-aa75-aa615fbb3465\"}]},\"type\":\"ConnectorPlacement.EquallySpacedConnector\",\"uuid\":\"bf69df94-f6ab-4503-8752-ba9a09e2aadb\"}],\"packageUris\":[\"http://schema.mathworks.com/mf0/Connector/R2020b\"],\"version\":\"1.0\"}"
  TEC_xxV Supply : Subsystem
      settings: PortSchema="{\"entries\":[{\"content\":{\"headerSize\":26,\"margin\":15,\"minimumSpacing\":25,\"sides\":[{\"content\":{\"connectorIds\":[]},\"type\":\"ConnectorPlacement.EquallySpacedRectSide\",\"uuid\":\"98751f74-1494-480e-afcb-1e4ca4833d8c\"},{\"content\":{\"connectorIds\":[],\"side\":\"RIGHT\"},\"type\":\"ConnectorPlacement.EquallySpacedRectSide\",\"uuid\":\"bb8add54-8697-4b5a-a683-6c55bc29b1b0\"},{\"content\":{\"connectorIds\":[\"Out1\"],\"side\":\"TOP\"},\"type\":\"ConnectorPlacement.EquallySpacedRectSide\",\"uuid\":\"300d0c82-b670-4163-bf95-251aaf6b9511\"},{\"content\":{\"connectorIds\":[],\"side\":\"BOTTOM\"},\"type\":\"ConnectorPlacement.EquallySpacedRectSide\",\"uuid\":\"167ec2d4-c810-4164-afac-a7cf55661aff\"}]},\"type\":\"ConnectorPlacement.EquallySpacedConnector\",\"uuid\":\"bf69df94-f6ab-4503-8752-ba9a09e2aadb\"}],\"packageUris\":[\"http://schema.mathworks.com/mf0/Connector/R2020b\"],\"version\":\"1.0\"}"
  Bus Element Out1 : Outport  PortName=120 VAC
  FBS1 : Outport  Port=2  PortName=FBS
  wires:
  TEC_xxV Supply/1(xxV) -> TEC Control Teensy/1(xxV)
  CMDS1/1 -> TEC Control Teensy/2(CMDS)
  TEC Control Teensy/1(FBS) -> FBS1/1

== system LFAST_System/INDI Client (PHD2 // KStars)/Plate Solver ==

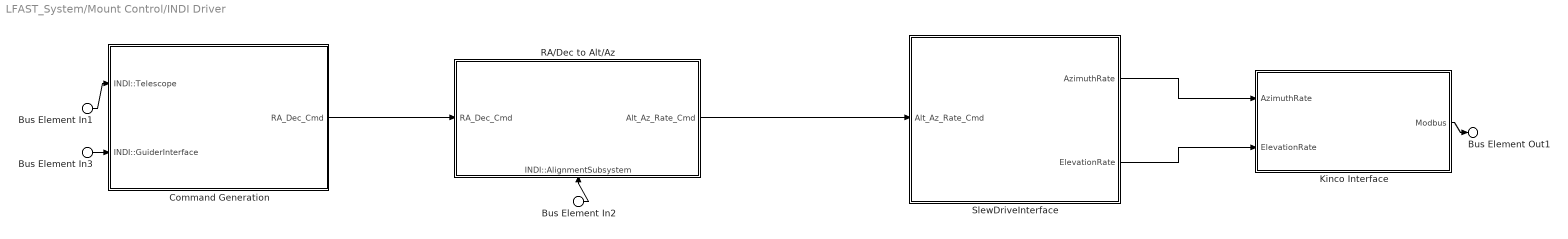
== system LFAST_System/Mount Control/INDI Driver ==
  Bus Element In1 : Inport  PortName=INDI::Telescope
  Bus Element In3 : Inport  Port=2  PortName=INDI::GuiderInterface
  Bus Element In2 : Inport  Port=3  PortName=INDI::AlignmentSubsystem
  Command Generation : Subsystem
      settings: PortSchema="{\"entries\":[{\"content\":{\"headerSize\":26,\"margin\":15,\"minimumSpacing\":25,\"sides\":[{\"content\":{\"connectorIds\":[\"In1\",\"In2\"]},\"type\":\"ConnectorPlacement.EquallySpacedRectSide\",\"uuid\":\"98751f74-1494-480e-afcb-1e4ca4833d8c\"},{\"content\":{\"connectorIds\":[\"Out1\"],\"side\":\"RIGHT\"},\"type\":\"ConnectorPlacement.EquallySpacedRectSide\",\"uuid\":\"bb8add54-8697-4b5a-a683-6c55bc29b1b0\"},{\"content\":{\"connectorIds\":[],\"side\":\"TOP\"},\"type\":\"ConnectorPlacement.EquallySpacedRectSide\",\"uuid\":\"300d0c82-b670-4163-bf95-251aaf6b9511\"}]},\"type\":\"ConnectorPlacement.EquallySpacedConnector\",\"uuid\":\"bf69df94-f6ab-4503-8752-ba9a09e2aadb\"}],\"packageUris\":[\"http://schema.mathworks.com/mf0/Connector/R2020b\"],\"version\":\"1.0\"}"
  Kinco Interface : Subsystem
      settings: PortSchema="{\"entries\":[{\"content\":{\"headerSize\":26,\"margin\":15,\"minimumSpacing\":25,\"sides\":[{\"content\":{\"connectorIds\":[\"In1\",\"In2\"]},\"type\":\"ConnectorPlacement.EquallySpacedRectSide\",\"uuid\":\"98751f74-1494-480e-afcb-1e4ca4833d8c\"},{\"content\":{\"connectorIds\":[\"Out1\"],\"side\":\"RIGHT\"},\"type\":\"ConnectorPlacement.EquallySpacedRectSide\",\"uuid\":\"bb8add54-8697-4b5a-a683-6c55bc29b1b0\"},{\"content\":{\"connectorIds\":[],\"side\":\"TOP\"},\"type\":\"ConnectorPlacement.EquallySpacedRectSide\",\"uuid\":\"300d0c82-b670-4163-bf95-251aaf6b9511\"}]},\"type\":\"ConnectorPlacement.EquallySpacedConnector\",\"uuid\":\"bf69df94-f6ab-4503-8752-ba9a09e2aadb\"}],\"packageUris\":[\"http://schema.mathworks.com/mf0/Connector/R2020b\"],\"version\":\"1.0\"}"
  RA/Dec to Alt/Az : Subsystem
      settings: PortSchema="{\"entries\":[{\"content\":{\"headerSize\":26,\"margin\":15,\"minimumSpacing\":25,\"sides\":[{\"content\":{\"connectorIds\":[\"In1\"]},\"type\":\"ConnectorPlacement.EquallySpacedRectSide\",\"uuid\":\"98751f74-1494-480e-afcb-1e4ca4833d8c\"},{\"content\":{\"connectorIds\":[\"Out1\"],\"side\":\"RIGHT\"},\"type\":\"ConnectorPlacement.EquallySpacedRectSide\",\"uuid\":\"bb8add54-8697-4b5a-a683-6c55bc29b1b0\"},{\"content\":{\"connectorIds\":[],\"side\":\"TOP\"},\"type\":\"ConnectorPlacement.EquallySpacedRectSide\",\"uuid\":\"300d0c82-b670-4163-bf95-251aaf6b9511\"},{\"content\":{\"connectorIds\":[\"In2\"],\"side\":\"BOTTOM\"},\"type\":\"ConnectorPlacement.EquallySpacedRectSide\",\"uuid\":\"ab0a47dd-fa3c-47e1-918e-dbc43bc49b36\"}]},\"type\":\"ConnectorPlacement.EquallySpacedConnector\",\"uuid\":\"bf69df94-f6ab-4503-8752-ba9a09e2aadb\"}],\"packageUris\":[\"http://schema.mathworks.com/mf0/Connector/R2020b\"],\"version\":\"1.0\"}"
  SlewDriveInterface : Subsystem
      settings: PortSchema="{\"entries\":[{\"content\":{\"headerSize\":26,\"margin\":15,\"minimumSpacing\":25,\"sides\":[{\"content\":{\"connectorIds\":[\"In1\"]},\"type\":\"ConnectorPlacement.EquallySpacedRectSide\",\"uuid\":\"98751f74-1494-480e-afcb-1e4ca4833d8c\"},{\"content\":{\"connectorIds\":[\"Out1\",\"Out2\"],\"side\":\"RIGHT\"},\"type\":\"ConnectorPlacement.EquallySpacedRectSide\",\"uuid\":\"bb8add54-8697-4b5a-a683-6c55bc29b1b0\"},{\"content\":{\"connectorIds\":[],\"side\":\"TOP\"},\"type\":\"ConnectorPlacement.EquallySpacedRectSide\",\"uuid\":\"300d0c82-b670-4163-bf95-251aaf6b9511\"}]},\"type\":\"ConnectorPlacement.EquallySpacedConnector\",\"uuid\":\"bf69df94-f6ab-4503-8752-ba9a09e2aadb\"}],\"packageUris\":[\"http://schema.mathworks.com/mf0/Connector/R2020b\"],\"version\":\"1.0\"}"
  Bus Element Out1 : Outport  PortName=Commands
  wires:
  Bus Element In2/1 -> RA/Dec to Alt/Az/2(INDI::AlignmentSubsystem)
  Bus Element In1/1 -> Command Generation/1(INDI::Telescope)
  Bus Element In3/1 -> Command Generation/2(INDI::GuiderInterface)
  Command Generation/1(RA_Dec_Cmd) -> RA/Dec to Alt/Az/1(RA_Dec_Cmd)
  RA/Dec to Alt/Az/1(Alt_Az_Rate_Cmd) -> SlewDriveInterface/1(Alt_Az_Rate_Cmd)
  SlewDriveInterface/1(AzimuthRate) -> Kinco Interface/1(AzimuthRate)
  SlewDriveInterface/2(ElevationRate) -> Kinco Interface/2(ElevationRate)
  Kinco Interface/1(Modbus) -> Bus Element Out1/1

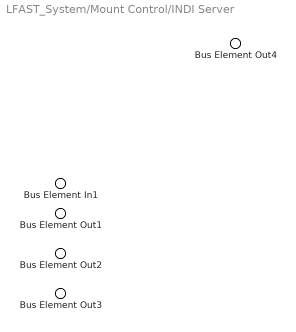
== system LFAST_System/Mount Control/INDI Server ==
  Bus Element In1 : Inport  PortName=INDI::MessageIn
  Bus Element Out4 : Outport  PortName=INDI::MessageOut
  Bus Element Out1 : Outport  Port=2  PortName=INDI::Telescope
  Bus Element Out2 : Outport  Port=3  PortName=INDI::GuiderInterface
  Bus Element Out3 : Outport  Port=4  PortName=INDI::AlignmentSubsystem

== system LFAST_System/Mount Control Box/Az Power Supply ==
  Bus Element Out1 : Outport  PortName=24V

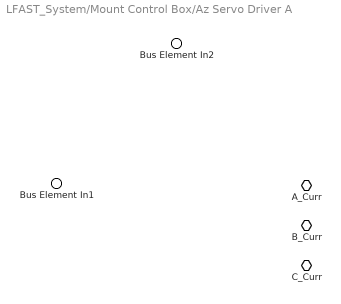
== system LFAST_System/Mount Control Box/Az Servo Driver A ==
  Bus Element In2 : Inport  PortName=CMDS
  Bus Element In1 : Inport  Port=2  PortName=24V
  A_Curr : PMIOPort  Side=Right
  B_Curr : PMIOPort  Port=2  Side=Right
  C_Curr : PMIOPort  Port=3  Side=Right

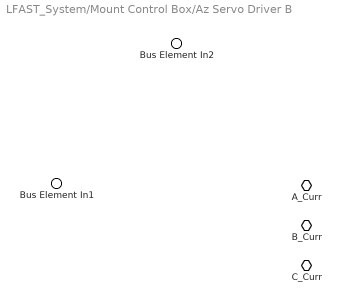
== system LFAST_System/Mount Control Box/Az Servo Driver B ==
  Bus Element In2 : Inport  PortName=CMDS
  Bus Element In1 : Inport  Port=2  PortName=24V
  A_Curr : PMIOPort  Side=Right
  B_Curr : PMIOPort  Port=2  Side=Right
  C_Curr : PMIOPort  Port=3  Side=Right

== system LFAST_System/Mount Control Box/El Power Supply ==
  Bus Element Out1 : Outport  PortName=24V

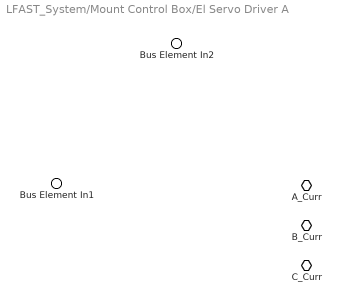
== system LFAST_System/Mount Control Box/El Servo Driver A ==
  Bus Element In2 : Inport  PortName=CMDS
  Bus Element In1 : Inport  Port=2  PortName=24V
  A_Curr : PMIOPort  Side=Right
  B_Curr : PMIOPort  Port=2  Side=Right
  C_Curr : PMIOPort  Port=3  Side=Right

== system LFAST_System/Mount Control Box/El Servo Driver B ==
  Bus Element In2 : Inport  PortName=CMDS
  Bus Element In1 : Inport  Port=2  PortName=24V
  A_Curr : PMIOPort  Side=Right
  B_Curr : PMIOPort  Port=2  Side=Right
  C_Curr : PMIOPort  Port=3  Side=Right

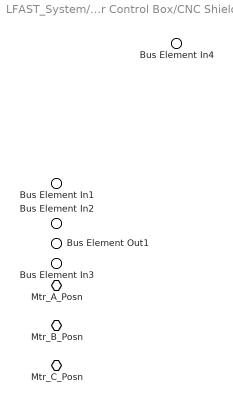
== system LFAST_System/Primary Mirror Control Box/CNC Shield ==
  Bus Element In4 : Inport  PortName=24V
  Bus Element In1 : Inport  Port=2  PortName=Mtr_A_Step
  Bus Element In2 : Inport  Port=3  PortName=Mtr_B_Step
  Bus Element In3 : Inport  Port=4  PortName=Mtr_C_Step
  Mtr_A_Posn : PMIOPort  Side=Right
  Mtr_B_Posn : PMIOPort  Port=2  Side=Right
  Mtr_C_Posn : PMIOPort  Port=3  Side=Right
  Bus Element Out1 : Outport  PortName=5V

== system LFAST_System/Primary Mirror Control Box/PMC_24V Supply ==
  Bus Element Out1 : Outport  PortName=24V

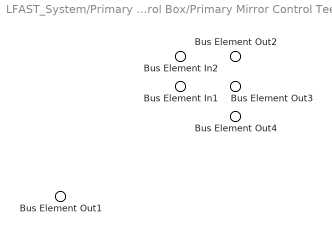
== system LFAST_System/Primary Mirror Control Box/Primary Mirror Control Teensy ==
  Bus Element In1 : Inport  PortName=5V
  Bus Element In2 : Inport  Port=2  PortName=CMDS
  Bus Element Out2 : Outport  PortName=Mtr_A_Step
  Bus Element Out3 : Outport  Port=2  PortName=Mtr_B_Step
  Bus Element Out4 : Outport  Port=3  PortName=Mtr_C_Step
  Bus Element Out1 : Outport  Port=4  PortName=FBS

== system LFAST_System/TEC Control Box/TEC Control Teensy ==
  Bus Element In3 : Inport  PortName=xxV
  Bus Element In1 : Inport  Port=2  PortName=CMDS
  Bus Element Out1 : Outport  PortName=FBS

== system LFAST_System/TEC Control Box/TEC_xxV Supply ==
  Bus Element Out1 : Outport  PortName=xxV

== system LFAST_System/Mount Control/INDI Driver/Command Generation ==
  Bus Element In1 : Inport  PortName=INDI::Telescope
  Bus Element In2 : Inport  Port=2  PortName=INDI::GuiderInterface
  Bus Element Out1 : Outport  PortName=RA_Dec_Cmd

== system LFAST_System/Mount Control/INDI Driver/Kinco Interface ==
  Bus Element In1 : Inport  PortName=AzimuthRate
  Bus Element In2 : Inport  Port=2  PortName=ElevationRate
  Bus Element Out1 : Outport  PortName=Modbus

== system LFAST_System/Mount Control/INDI Driver/RA//Dec to Alt//Az ==
  Bus Element In2 : Inport  PortName=RA_Dec_Cmd
  Bus Element In1 : Inport  Port=2  PortName=INDI::AlignmentSubsystem
  Bus Element Out1 : Outport  PortName=Alt_Az_Rate_Cmd

== system LFAST_System/Mount Control/INDI Driver/SlewDriveInterface ==
  Bus Element In1 : Inport  PortName=Alt_Az_Rate_Cmd
  Bus Element Out1 : Outport  PortName=AzimuthRate
  Bus Element Out2 : Outport  Port=2  PortName=ElevationRate
